simulink model "Predefined_with_GroundTruth_mod1acc"  (R2021b)
settings: Solver=VariableStepAuto  StartTime=0.0  StopTime=inf  RelTol=1e-3
model workspace (MAT data in the model file):
  firstWarning = 1
  originalScenarioChecksum = '114339432DE22364D47BB28FC96DC10C'
undefined symbols (not defined in the file or in its folder): Acceleration, ActorID, AngularVelocity, curvature, curvatureAhd, DefaultGear, DEND_B, DEND_S, DEND_T, direction, driving, gradbp, LF, LR, matlabshared, MAX_BRAKE, MAX_STEER, MAX_TORQUE, MCAR, MIN_BRAKE, MIN_STEER, MIN_TORQUE, NUMD_B, NUMD_S, NUMD_T, Pitch, Position, psi_o, R, Roll, RRdamp, scenario, SceneInfo, sigbuilder_block, STEER_RATIO, stopSign_ID, Tdead, thetaRefs, TL_ID, TrackWidth, Ts, ts, Vdead, Velocity, X_o, xRef2s, Y_o, Yaw, yRef2s
libraries: mpcsigdimcheck_private x10, drivingscenarioandsensors x8, drivingvehiclecontroller x2, slpidlib x2, simulink x2, trackingutilitieslib x2, mpclib x1, simulink_extras x1, drivinglib x1, autolibshared x1, vehdynlibviscommon x1, vehdynlibsteering x1
(part 2 of 3)

== system Predefined_with_GroundTruth_mod1acc/Tracking/Subsystem1 ==
  In2 : Inport
  EgoV : Inport  Port=2
  Camera : drivingscenarioandsensors/Vision Detection Generator  SensorIndex=1  DetectorOutput=Objects only  UpdateInterval=0.1  LaneUpdateInterval=0.1  SensorLocation=[1.9 0]  Height=1.1  Yaw=0  Pitch=1  Roll=0  BusNameSource=Auto  BusName=BusObjectDetections  BusName2Source=Auto  BusName2=BusLaneDetections  MaxNumDetectionsSource=Property  MaxNumDetections=10  MaxNumLanesSource=Property  MaxNumLanes=30  DetectionCoordinates=Ego Cartesian  SimulateUsing=Interpreted execution  MaxRange=150  BoundingBoxAccuracy=5  ProcessNoiseIntensity=5  MaxSpeed=100  MaxAllowedOcclusion=0.5  MinObjectImageSize=[5 5]  DetectionProbability=0.9  FalsePositivesPerImage=0.1  MinLaneImageSize=[20 3]  LaneBoundaryAccuracy=3  HasNoise=on  InitialSeedSource=Repeatable  InitialSeed=0  UsedSeed=0  ActorProfilesSource=From Scenario Reader block  ActorProfilesParameters=driving.internal.ActorProfilesParameters  ActorProfilesExpression=[struct('ActorID',1,'ClassID',1,'Length',4.7,'Width',1.8,'Height',1.4,'OriginOffset',[-1.35 0 0],'MeshVertices',[3.7 0.9 0.857439446366782;3.7 -0.9 0.857439446366782;3.7 -0.9 0.314878892733564;3.7 0.9 0.314878892733564;3.7 0.9 0.857439446366782;2.525 0.9 0.993079584775086;2.525 -0.9 0.993079584775086;3.7 -0.9 0.857439446366782;1.82 0.72 1.4;0.41 0.72 1.4;0.41 -0.72 1.4;1.82 -0.72 1.4;-0.295 0.9 0.993079584775086;-1 0.9 0.857439446366782;-1 -0.9 0.857439446366782;-0.295 -0.9 0.993079584775086;3.7 0.9 0.857439446366782;3.7 0.9 0.314878892733564;2.525 0.9 0.314878892733564;2.525 0.9 0.993079584775086;2.525 0.9 0.993079584775086;2.525 0.9 0.314878892733564;-0.295 0.9 0.314878892733564;-0.295 0.9 0.993079584775086;-0.295 0.9 0.993079584775086;-0.295 0.9 0.314878892733564;-1 0.9 0.355570934256055;-1 0.9 0.857439446366782;2.525 0.9 0.993079584775086;-0.295 0.9 0.993079584775086;0.41 0.72 1.4;1.82 0.72 1.4;3.7 -0.9 0.857439446366782;3.7 -0.9 0.314878892733564;2.525 -0.9 0.314878892733564;2.525 -0.9 0.993079584775086;2.525 -0.9 0.993079584775086;2.525 -0.9 0.314878892733564;-0.295 -0.9 0.314878892733564;-0.295 -0.9 0.993079584775086;-0.295 -0.9 0.993079584775086;-0.295 -0.9 0.314878892733564;-1 -0.9 0.355570934256055;-1 -0.9 0.857439446366782;2.525 -0.9 0.993079584775086;-0.295 -0.9 0.993079584775086;0.41 -0.72 1.4;1.82 -0.72 1.4;-0.295 0.9 0.993079584775086;-0.295 -0.9 0.993079584775086;0.41 -0.72 1.4;0.41 0.72 1.4;2.525 -0.9 0.993079584775086;1.82 -0.72 1.4;1.82 0.72 1.4;2.525 0.9 0.993079584775086;-1 0.9 0.857439446366782;-1 0.9 0.355570934256055;-1 -0.9 0.355570934256055;-1 -0.9 0.857439446366782;3.7 0.9 0.314878892733564;3.7 -0.9 0.314878892733564;-0.295 -0.9 0.314878892733564;-0.295 0.9 0.314878892733564;-0.295 0.9 0.314878892733564;-1 0.9 0.355570934256055;-1 -0.9 0.355570934256055;-0.295 -0.9 0.314878892733564;0 -0.63 0;0 -0.87 0;0.191030206995054 -0.63 0.0601365173421445;0.191030206995054 -0.87 0.0601365173421445;0.309093367795925 -0.63 0.217575963708927;0.309093367795925 -0.87 0.217575963708927;0.309093367795925 -0.63 0.412181821758201;0.309093367795925 -0.87 0.412181821758201;0.191030206995054 -0.63 0.569621268124983;0.191030206995054 -0.87 0.569621268124983;0 -0.63 0.629757785467128;0 -0.87 0.629757785467128;-0.191030206995054 -0.63 0.569621268124983;-0.191030206995054 -0.87 0.569621268124983;-0.309093367795925 -0.63 0.412181821758201;-0.309093367795925 -0.87 0.412181821758201;-0.309093367795925 -0.63 0.217575963708927;-0.309093367795925 -0.87 0.217575963708927;-0.191030206995054 -0.63 0.0601365173421445;-0.191030206995054 -0.87 0.0601365173421445;0 -0.63 0;0 -0.87 0;0 -0.63 0;0.191030206995054 -0.63 0.0601365173421445;0.309093367795925 -0.63 0.217575963708927;0.309093367795925 -0.63 0.412181821758201;0.191030206995054 -0.63 0.569621268124983;0 -0.63 0.629757785467128;-0.191030206995054 -0.63 0.569621268124983;-0.309093367795925 -0.63 0.412181821758201;-0.309093367795925 -0.63 0.217575963708927;-0.191030206995054 -0.63 0.0601365173421445;0 -0.87 0;0.191030206995054 -0.87 0.0601365173421445;0.309093367795925 -0.87 0.217575963708927;0.309093367795925 -0.87 0.412181821758201;0.191030206995054 -0.87 0.569621268124983;0 -0.87 0.629757785467128;-0.191030206995054 -0.87 0.569621268124983;-0.309093367795925 -0.87 0.412181821758201;-0.309093367795925 -0.87 0.217575963708927;-0.191030206995054 -0.87 0.0601365173421445;0 0.87 0;0 0.63 0;0.191030206995054 0.87 0.0601365173421445;0.191030206995054 0.63 0.0601365173421445;0.309093367795925 0.87 0.217575963708927;0.309093367795925 0.63 0.217575963708927;0.309093367795925 0.87 0.412181821758201;0.309093367795925 0.63 0.412181821758201;0.191030206995054 0.87 0.569621268124983;0.191030206995054 0.63 0.569621268124983;0 0.87 0.629757785467128;0 0.63 0.629757785467128;-0.191030206995054 0.87 0.569621268124983;-0.191030206995054 0.63 0.569621268124983;-0.309093367795925 0.87 0.412181821758201;-0.309093367795925 0.63 0.412181821758201;-0.309093367795925 0.87 0.217575963708927;-0.309093367795925 0.63 0.217575963708927;-0.191030206995054 0.87 0.0601365173421445;-0.191030206995054 0.63 0.0601365173421445;0 ...(+3718 chars)],'MeshFaces',[1 2 3;3 4 1;5 6 7;7 8 5;9 10 11;11 12 9;13 14 15;15 16 13;17 18 19;19 20 17;21 22 23;23 24 21;25 26 27;27 28 25;29 30 31;31 32 29;33 34 35;35 36 33;37 38 39;39 40 37;41 42 43;43 44 41;45 46 47;47 48 45;49 50 51;51 52 49;53 54 55;55 56 53;57 58 59;59 60 57;61 62 63;63 64 61;65 66 67;67 68 65;69 71 72;72 70 69;71 73 74;74 72 71;73 75 76;76 74 73;75 77 78;78 76 75;77 79 80;80 78 77;79 81 82;82 80 79;81 83 84;84 82 81;83 85 86;86 84 83;85 87 88;88 86 85;87 89 90;90 88 87;91 92 93;91 93 94;91 94 95;91 95 96;91 96 97;91 97 98;91 98 99;91 99 100;101 102 103;101 103 104;101 104 105;101 105 106;101 106 107;101 107 108;101 108 109;101 109 110;111 113 114;114 112 111;113 115 116;116 114 113;115 117 118;118 116 115;117 119 120;120 118 117;119 121 122;122 120 119;121 123 124;124 122 121;123 125 126;126 124 123;125 127 128;128 126 125;127 129 130;130 128 127;129 131 132;132 130 129;133 134 135;133 135 136;133 136 137;133 137 138;133 138 139;133 139 140;133 140 141;133 141 142;143 144 145;143 145 146;143 146 147;143 147 148;143 148 149;143 149 150;143 150 151;143 151 152;153 155 156;156 154 153;155 157 158;158 156 155;157 159 160;160 158 157;159 161 162;162 160 159;161 163 164;164 162 161;163 165 166;166 164 163;165 167 168;168 166 165;167 169 170;170 168 167;169 171 172;172 170 169;171 173 174;174 172 171;175 176 177;175 177 178;175 178 179;175 179 180;175 180 181;175 181 182;175 182 183;175 183 184;185 186 187;185 187 188;185 188 189;185 189 190;185 190 191;185 191 192;185 192 193;185 193 194;195 197 198;198 196 195;197 199 200;200 198 197;199 201 202;202 200 199;201 203 204;204 202 201;203 205 206;206 204 203;205 207 208;208 206 205;207 209 210;210 208 207;209 211 212;212 210 209;211 213 214;214 212 211;213 215 216;216 214 213;217 218 219;217 219 220;217 220 221;217 221 222;217 222 223;217 223 224;217 224 225;217 225 226;227 228 229;227 229 230;227 230 231;227 231 232;227 232 233;227 233 234;227 234 235;227 235 236],'RCSPattern',[10 10;10 10],'RCSAzimuthAngles',[-180 180],'RCSElevationAngles',[-90 90]); struct('ActorID',2,'ClassID',7,'Length',0.7,'Width',0.2,'Height',0.1,'OriginOffset',[0 0 0],'MeshVertices',[0.35 -0.1 0.1;0.35 0.1 0.1;-0.35 0.1 0.1;-0.35 -0.1 0.1;0.35 -0.1 0;0.35 0.1 0;-0.35 0.1 0;-0.35 -0.1 0],'MeshFaces',[6 2 1;1 5 6;8 4 3;3 7 8;6 7 3;3 2 6;5 1 4;4 8 5;4 1 2;2 3 4;7 6 5;5 8 7],'RCSPattern',[10 10;10 10],'RCSAzimuthAngles',[-180 180],'RCSElevationAngles',[-90 90])]  Intrinsics=driving.internal.cameraIntrinsics('FocalLength',[800 800],'PrincipalPoint',[320 240],'ImageSize',[480 640],'RadialDistortion',[0 0],'TangentialDistortion',[0 0],'Skew',0)
  Detection Concatenation : trackingutilitieslib/Detection Concatenation  NumInputs=3  BusNameSource=Auto  BusName=BusDetectionConcatenation  SimulateUsing=Interpreted execution
      settings: SourceProductBaseCode=AE,DR,TF,RA,UV,VE
  Lidar Point Cloud Generator : drivingscenarioandsensors/Lidar Point Cloud Generator  SensorIndex=2  UpdateInterval=0.1  SensorLocation=[1.5 0]  Height=1.6  Yaw=0  Pitch=0  Roll=0  DetectionCoordinates=Ego Cartesian  HasEgoVehicle=on  EgoVehicleActorID=1  HasRoadsInputPort=on  ActorProfilesSource=From Scenario Reader block  ActorProfilesVariableName=actor_profiles  MaxRange=120  RangeAccuracy=0.002  AzimuthResolution=0.16  ElevationResolution=1.25  AzimuthLimits=[-60 60]  ElevationLimits=[ -20, 20 ]  HasNoise=on
      settings: SourceProductBaseCode=DR
  Lidar Point Cloud Generator1 : drivingscenarioandsensors/Lidar Point Cloud Generator  SensorIndex=3  UpdateInterval=0.1  SensorLocation=[1.5 0]  Height=1.6  Yaw=0  Pitch=0  Roll=0  DetectionCoordinates=Ego Cartesian  HasEgoVehicle=on  EgoVehicleActorID=1  HasRoadsInputPort=on  ActorProfilesSource=From Scenario Reader block  ActorProfilesVariableName=actor_profiles  MaxRange=120  RangeAccuracy=0.002  AzimuthResolution=0.16  ElevationResolution=1.25  AzimuthLimits=[60 180]  ElevationLimits=[ -20, 20 ]  HasNoise=on
      settings: SourceProductBaseCode=DR
  Lidar Point Cloud Generator2 : drivingscenarioandsensors/Lidar Point Cloud Generator  SensorIndex=4  UpdateInterval=0.1  SensorLocation=[1.5 0]  Height=1.6  Yaw=0  Pitch=0  Roll=0  DetectionCoordinates=Ego Cartesian  HasEgoVehicle=on  EgoVehicleActorID=1  HasRoadsInputPort=on  ActorProfilesSource=From Scenario Reader block  ActorProfilesVariableName=actor_profiles  MaxRange=120  RangeAccuracy=0.002  AzimuthResolution=0.16  ElevationResolution=1.25  AzimuthLimits=[-180 -60]  ElevationLimits=[ -20, 20 ]  HasNoise=on
      settings: SourceProductBaseCode=DR
  Camera Detections : Outport
  Radar detections : Outport  Port=2
  wires:
  EgoV/1 -> Lidar Point Cloud Generator1/2, Lidar Point Cloud Generator/2, Lidar Point Cloud Generator2/2
  Lidar Point Cloud Generator1/1 -> Detection Concatenation/2  "Lidar Detections"
  Lidar Point Cloud Generator2/1 -> Detection Concatenation/3  "Lidar Detections"
  Detection Concatenation/1 -> Radar detections/1
  Camera/1 -> Camera Detections/1  "Camera Detections"
  In2/1 -> Camera/1, Lidar Point Cloud Generator/1, Lidar Point Cloud Generator1/1, Lidar Point Cloud Generator2/1
  Lidar Point Cloud Generator/1 -> Detection Concatenation/1  "Lidar Detections"

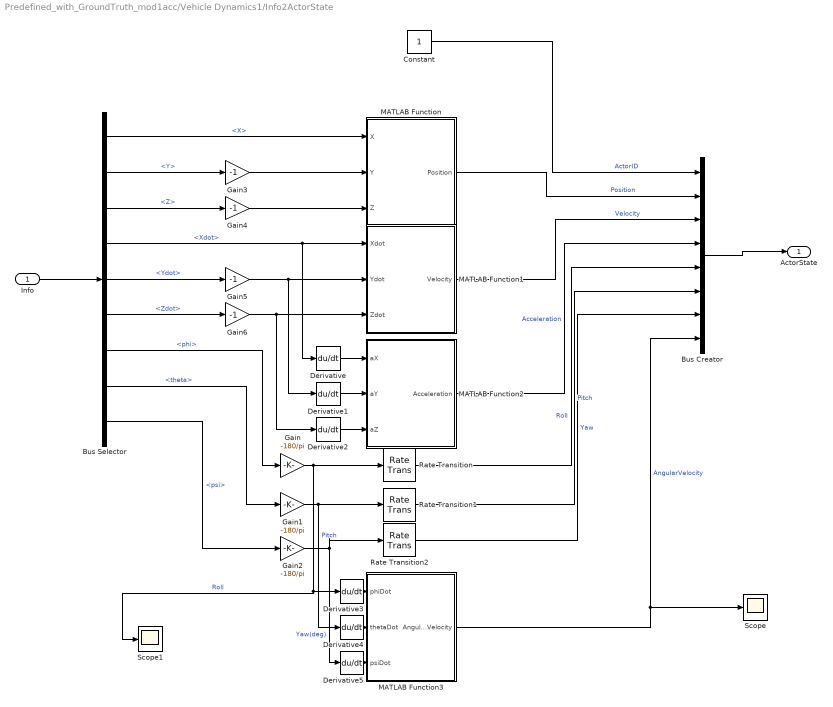
== system Predefined_with_GroundTruth_mod1acc/Vehicle Dynamics1/Info2ActorState ==
  Info : Inport
  Bus Creator : BusCreator  Inputs=ActorID,Position,Velocity,Acceleration,Roll,Pitch,Yaw,AngularVelocity  OutDataTypeStr=Bus: BusActorState  NonVirtualBus=on
  Bus Selector : BusSelector  OutputSignals=InertFrm.Cg.Disp.X,InertFrm.Cg.Disp.Y,InertFrm.Cg.Disp.Z,InertFrm.Cg.Vel.Xdot,InertFrm.Cg.Vel.Ydot,InertFrm.Cg.Vel.Zdot,InertFrm.Cg.Ang.phi,InertFrm.Cg.Ang.theta,InertFrm.Cg.Ang.psi
  Constant : Constant  SampleTime=0.05
  Derivative{,1..5} (6 alike) : Derivative
  Gain : Gain  Gain=-180/pi
  Gain1 : Gain  Gain=-180/pi
  Gain2 : Gain  Gain=-180/pi
  Gain{3..6} (4 alike) : Gain  Gain=-1
  MATLAB Function : MATLAB Function  TreatAsAtomicUnit=on  SystemSampleTime=0.05
  MATLAB Function1 : MATLAB Function  TreatAsAtomicUnit=on  SystemSampleTime=0.05
  MATLAB Function2 : MATLAB Function  TreatAsAtomicUnit=on  SystemSampleTime=0.05
  MATLAB Function3 : MATLAB Function  TreatAsAtomicUnit=on  SystemSampleTime=0.05
  Rate Transition : RateTransition  OutPortSampleTime=0.05
  Rate Transition1 : RateTransition  OutPortSampleTime=0.05
  Rate Transition2 : RateTransition  OutPortSampleTime=0.05
  Scope : Scope
  Scope1 : Scope
  ActorState : Outport
  wires:
  Gain/1 -> Scope1/1, Derivative3/1, Rate Transition/1  "Roll"
  Derivative4/1 -> MATLAB Function3/2(thetaDot)
  Bus Selector/2 -> Gain3/1  "<Y>"
  Bus Selector/4 -> Derivative/1, MATLAB Function1/1(Xdot)  "<Xdot>"
  MATLAB Function1/1(Velocity) -> Bus Creator/3  "Velocity"
  MATLAB Function/1(Position) -> Bus Creator/2  "Position"
  Derivative1/1 -> MATLAB Function2/2(aY)
  Bus Selector/5 -> Gain5/1  "<Ydot>"
  Bus Selector/1 -> MATLAB Function/1(X)  "<X>"
  Bus Selector/9 -> Gain2/1  "<psi>"
  Gain2/1 -> Rate Transition2/1, Derivative5/1  "Yaw(deg)"
  Derivative5/1 -> MATLAB Function3/3(psiDot)
  Bus Selector/7 -> Gain/1  "<phi>"
  MATLAB Function2/1(Acceleration) -> Bus Creator/4  "Acceleration"
  Derivative3/1 -> MATLAB Function3/1(phiDot)
  Gain1/1 -> Derivative4/1, Rate Transition1/1  "Pitch"
  Bus Selector/6 -> Gain6/1  "<Zdot>"
  Bus Selector/8 -> Gain1/1  "<theta>"
  MATLAB Function3/1(AngularVelocity) -> Bus Creator/8, Scope/1  "AngularVelocity"
  Bus Selector/3 -> Gain4/1  "<Z>"
  Derivative2/1 -> MATLAB Function2/3(aZ)
  Derivative/1 -> MATLAB Function2/1(aX)
  Info/1 -> Bus Selector/1
  Constant/1 -> Bus Creator/1  "ActorID"
  Bus Creator/1 -> ActorState/1
  Rate Transition/1 -> Bus Creator/5  "Roll"
  Rate Transition1/1 -> Bus Creator/6  "Pitch"
  Rate Transition2/1 -> Bus Creator/7  "Yaw"
  Gain3/1 -> MATLAB Function/2(Y)
  Gain4/1 -> MATLAB Function/3(Z)
  Gain5/1 -> Derivative1/1, MATLAB Function1/2(Ydot)
  Gain6/1 -> Derivative2/1, MATLAB Function1/3(Zdot)

== system Predefined_with_GroundTruth_mod1acc/Vehicle Dynamics1/Subsystem ==
  Gain : Gain  Gain=MAX_TORQUE*0.1
  Gain1 : Gain  Gain=MIN_BRAKE*0.06
  Gain2 : Gain  Gain=MAX_STEER/4.5
  Signal Builder : Subsystem  Tag=STV Subsys  LoadFcn=sigbuilder_block('load');  StartFcn=sigbuilder_block('start');  StopFcn=sigbuilder_block('stop');  ClipboardFcn=sigbuilder_block('clipboard');  mask(Sigbuilder block){tuvar=[0:10]}
      mask help: Simulink:masks:SigbuilderBlock_MD
      mask init:
      | if ~strcmp(get_param(bdroot(gcbh),'SimulationStatus'),'stopped') tuvar = sigbuilder_block('maskInit'); end
      settings: CopyFcn=sigbuilder_block('copy');  DeleteFcn=sigbuilder_block('delete');  ModelCloseFcn=sigbuilder_block('modelClose');  PreSaveFcn=sigbuilder_block('preSave');  PauseFcn=sigbuilder_block('pause');  ContinueFcn=sigbuilder_block('continue');  NameChangeFcn=sigbuilder_block('namechange');  OpenFcn=sigbuilder_block('open',[0 30 960 455.5 ]);  CloseFcn=sigbuilder_block('close');
      mask Display: plot(0, 0, 100, 100,[2, 2, 32, 32, 2], [68, 8, 8, 68, 68],[32, 2], [38, 38], [32, 19, 2],[53, 60, 44], [32, 17, 17, 2],[16, 16, 31, 31]);txt = getActiveGroup(gcbh);text(2, 100, txt,'verticalAlignment', 'top');
  torque_cmd (Nm) : Outport
  brake_cmd (Nm) : Outport  Port=2
  steer_cmd (deg) : Outport  Port=3
  wires:
  Gain2/1 -> steer_cmd (deg)/1  "steer_cmd (deg)"
  Signal Builder/1(Normalized Torque) -> Gain/1
  Signal Builder/2(Normalized Brake) -> Gain1/1
  Signal Builder/3(Normalized Steer) -> Gain2/1  "steer_cmd (deg)"
  Gain1/1 -> brake_cmd (Nm)/1  "brake_cmd (Nm)"
  Gain/1 -> torque_cmd (Nm)/1  "torque_cmd (Nm)"

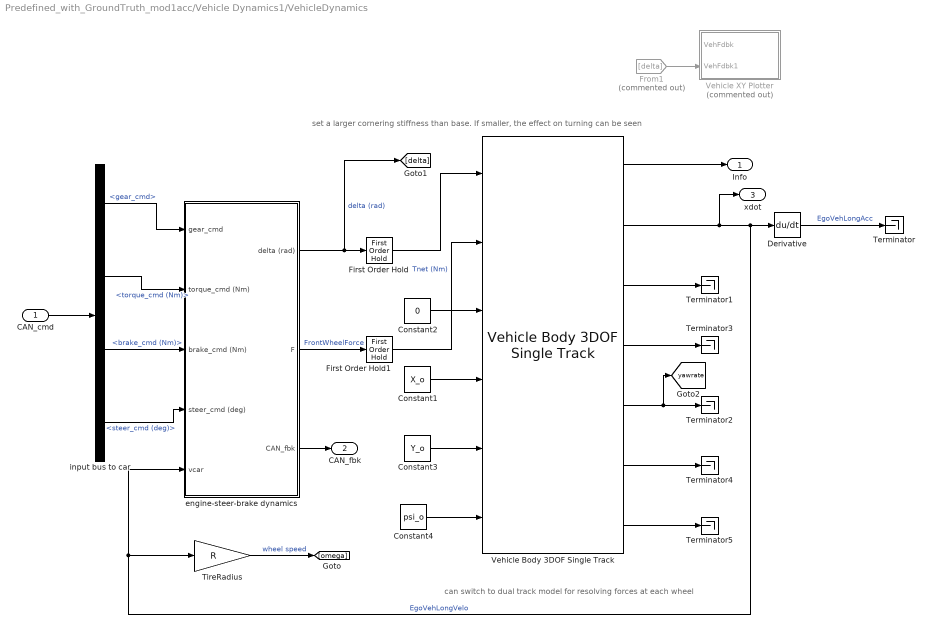
== system Predefined_with_GroundTruth_mod1acc/Vehicle Dynamics1/VehicleDynamics ==
  note: set a larger cornering stiffness than base. If smaller, the effect on turning can be seen
  note: can switch to dual track model for resolving forces at each wheel
  CAN_cmd : Inport
  Constant1 : Constant  Value=X_o
  Constant2 : Constant  Value=0
  Constant3 : Constant  Value=Y_o
  Constant4 : Constant  Value=psi_o
  Derivative : Derivative
  First Order Hold : FirstOrderHold  ErrorTolerance=inf
  First Order Hold1 : FirstOrderHold  ErrorTolerance=inf
  From1 : From  Commented=on  GotoTag=delta
  Terminator{,1..5} (6 alike) : Terminator
  TireRadius : Gain  Gain=R
  Vehicle Body 3DOF Single Track : autolibshared/Vehicle Body 3DOF Single Track  trackMode=Single (bicycle)  inputMode=External longitudinal forces  frontSteerMode=on  rearSteerMode=off  windMode=off  muMode=off  extFMode=off  extMMode=off  htchFMode=off  htchMMode=off  extXo=on  extpsio=on  extxdoto=off  extro=off  extYo=on  extTamb=off  extydoto=off  aMode=2  NF=2  NR=2  m=MCAR  a=LF  b=LR  h=0.35  dh=1  hh=0.2  X_o=InitPosition(1)  xdot_o=InitSpeed  CalphaMode=off  sigmaMode=on  d=0  hl=0  w=[1.4,1.4]  Cy_f=12e3*100  Cy_r=11e3*100  sigma_f=.1  sigma_r=.1  alpha_f_brk=[-.1 .1]  Cy_f_data=[-9e3 9e3]  alpha_r_brk=[-.1 .1]  Cy_r_data=[-9e3 9e3]  Y_o=-InitPosition(2)  ydot_o=0  Izz=2050  psi_o=-InitYaw/180*pi  r_o=0  Af=2  Cd=.3  Cl=.1  Cpm=.1  beta_w=[0:0.01:0.3]  Cs=[0:0.03:0.9]  Cym=[0:0.01:0.3]  Pabs=101325  Tair=273  g=9.81  mu=1  xdot_tol=.01  Fznom=5000  Fxtire_sat=7e4  Fytire_sat=7e4  longOff=0  latOff=0  vertOff=0  wrapAng=off
      settings: SourceProductBaseCode=PW,DR,MT,UV,VE
  Vehicle XY Plotter : Subsystem  Commented=on  mask(Vehicle XY Plotter){a=LF, b=LR, w=TrackWidth, bufferSize=1024, pltDT=.1}
      mask prompts: a "Distance to front axle from CG, a [m]:"; b "Distance to rear axle from CG, b [m]:"; w "Track width, w [m]:"; bufferSize "Path buffer sampe size, bufferSize []:"; pltDT "Plot update rate, pltDT [s]:"
      mask help: This block will display a MATLAB figure which indicates the vehicle path, current position and heading velocity.
      mask TypeOptions a: Vehicle XY Plotter/a
      mask TypeOptions b: Vehicle XY Plotter/b
      mask TypeOptions w: Vehicle XY Plotter/w
      mask TypeOptions bufferSize: Vehicle XY Plotter/bufferSize
  engine-steer-brake dynamics : Subsystem
  input bus to car : BusSelector  OutputSignals=gear_cmd,torque_cmd (Nm),brake_cmd (Nm),steer_cmd (deg)
  Info : Outport
  CAN_fbk : Outport  Port=2  VectorParamsAs1DForOutWhenUnconnected=off
  xdot : Outport  Port=3
  tag scope: yawrate=global
  wires:
  TireRadius/1 -> [omega]  "wheel speed"
  Vehicle Body 3DOF Single Track/1 -> Info/1
  From1/1 -> Vehicle XY Plotter/2(VehFdbk1)
  input bus to car/1 -> engine-steer-brake dynamics/1(gear_cmd)  "<gear_cmd>"
  input bus to car/3 -> engine-steer-brake dynamics/3(brake_cmd (Nm))  "<brake_cmd (Nm)>"
  engine-steer-brake dynamics/1(delta (rad)) -> [delta], First Order Hold/1  "delta (rad)"
  input bus to car/2 -> engine-steer-brake dynamics/2(torque_cmd (Nm))  "<torque_cmd (Nm)>"
  input bus to car/4 -> engine-steer-brake dynamics/4(steer_cmd (deg))  "<steer_cmd (deg)>"
  engine-steer-brake dynamics/3(CAN_fbk) -> CAN_fbk/1
  CAN_cmd/1 -> input bus to car/1
  Constant2/1 -> Vehicle Body 3DOF Single Track/3
  engine-steer-brake dynamics/2(F) -> First Order Hold1/1  "FrontWheelForce"
  First Order Hold/1 -> Vehicle Body 3DOF Single Track/1
  Vehicle Body 3DOF Single Track/2 -> xdot/1, engine-steer-brake dynamics/5(vcar), TireRadius/1, Derivative/1  "EgoVehLongVelo"
  Vehicle Body 3DOF Single Track/3 -> Terminator1/1
  Vehicle Body 3DOF Single Track/4 -> Terminator3/1
  Vehicle Body 3DOF Single Track/5 -> [yawrate], Terminator2/1
  Vehicle Body 3DOF Single Track/6 -> Terminator4/1
  Vehicle Body 3DOF Single Track/7 -> Terminator5/1
  Derivative/1 -> Terminator/1  "EgoVehLongAcc"
  First Order Hold1/1 -> Vehicle Body 3DOF Single Track/2  "Tnet (Nm)"
  Constant1/1 -> Vehicle Body 3DOF Single Track/4
  Constant3/1 -> Vehicle Body 3DOF Single Track/5
  Constant4/1 -> Vehicle Body 3DOF Single Track/6

== system Predefined_with_GroundTruth_mod1acc/Reference Data/Theta/thetaBlocks ==
  note: theta calculated from Simulink blocks
  y : Inport
  x : Inport  Port=2
  dis : Inport  Port=3
  Atan2 : Trigonometry  Operator=atan2  ApproximationMethod=CORDIC
  Difference : simulink/Discrete/Difference  ICPrevInput=0.0  OutMin=[]  OutMax=[]  OutDataType=fixdt(1, 16)  OutScaling=2^-10  DoSatur=off
  Difference1 : simulink/Discrete/Difference  ICPrevInput=0.0  OutMin=[]  OutMax=[]  OutDataType=fixdt(1, 16)  OutScaling=2^-10  DoSatur=off
  IC : InitialCondition  Value=psi_o
  Radians to Degrees : simulink_extras/Transformations/Radians to Degrees
  Terminator : Terminator
  theta : Outport
  wires:
  IC/1 -> Radians to Degrees/1
  Atan2/1 -> IC/1
  dis/1 -> Terminator/1
  x/1 -> Difference1/1
  y/1 -> Difference/1
  Radians to Degrees/1 -> theta/1
  Difference/1 -> Atan2/1
  Difference1/1 -> Atan2/2

== system Predefined_with_GroundTruth_mod1acc/Reference Data/Theta/thetaLt ==
  note: Check out the script "setUpModel" to understand how we have calculated theta
  note: theta based on lookup table
  y : Inport
  x : Inport  Port=2
  dis : Inport  Port=3
  Terminator : Terminator
  Terminator1 : Terminator
  Theta Ref : Lookup_n-D  NumberOfTableDimensions=1  BreakpointsForDimension1=gradbp  Table=thetaRefs  InternalRulePriority=Speed  RndMeth=Simplest  InputSameDT=on
  theta : Outport
  wires:
  Theta Ref/1 -> theta/1
  dis/1 -> Theta Ref/1
  x/1 -> Terminator1/1
  y/1 -> Terminator/1

== system Predefined_with_GroundTruth_mod1acc/Subsystem3/Subsystem1/Subsystem2 ==
  acc_cmd : Inport
  decc_cmd : Inport  Port=2
  Subsystem : Subsystem
  Subsystem1 : Subsystem
  T_eng_cmd : Outport
  brake_cmd : Outport  Port=2
  wires:
  acc_cmd/1 -> Subsystem/1(acc_cmd)
  Subsystem/1(T_eng_cmd) -> T_eng_cmd/1
  decc_cmd/1 -> Subsystem1/1(decc_cmd)
  Subsystem1/1(T_brake_cmd) -> brake_cmd/1

== system Predefined_with_GroundTruth_mod1acc/Subsystem3/Subsystem2/Subsystem2 ==
  acc_cmd : Inport
  decc_cmd : Inport  Port=2
  Subsystem : Subsystem
  Subsystem1 : Subsystem
  T_eng_cmd : Outport
  brake_cmd : Outport  Port=2
  wires:
  acc_cmd/1 -> Subsystem/1(acc_cmd)
  Subsystem/1(T_eng_cmd) -> T_eng_cmd/1
  decc_cmd/1 -> Subsystem1/1(decc_cmd)
  Subsystem1/1(T_brake_cmd) -> brake_cmd/1

== system Predefined_with_GroundTruth_mod1acc/Vehicle Dynamics1/Subsystem/Signal Builder ==
  Demux : Demux  Tag=STV Demux  Outputs=3
      settings: DisplayOption=none
  FromWs : FromWorkspace  Tag=STV FromWs  VariableName=tuvar
      SigBuilderData=|
      | common.afterFinalStr = 'Extrapolate'
      | common.sampleTime = 0
      | dataSet.timeRange = [0 3.5]
      | dataSet.name = 'DriveAndTurn'
      | sbobj.Groups.Name = 'DriveAndTurn'
      | sbobj.Groups.Signals(1).Name = 'Normalized Torque'
      | sbobj.Groups.Signals(1).XData = [0 1 1 2 2 3.5]
      | sbobj.Groups.Signals(1).YData = [1 1 0 0 1 1]
      | sbobj.Groups.Signals(2).Name = 'Normalized Brake'
      | sbobj.Groups.Signals(2).XData = [0 1 1 2 2 3.5]
      | sbobj.Groups.Signals(2).YData = [0 0 1 1 0 0]
      | sbobj.Groups.Signals(3).Name = 'Normalized Steer'
      | sbobj.Groups.Signals(3).XData = [0 0.5 0.6 1.02 1.02 2 2.5 3 3.5]
      | sbobj.Groups.Signals(3).YData = [-0.02 -0.02 -0.02 -0.3 -1.02 -0.92 -0.34 0.14 0.22]
      | sbobj.Groups.TimeRange = [0 3.5]
  Normalized Torque : Outport  Tag=STV Outport
  Normalized Brake : Outport  Tag=STV Outport  Port=2
  Normalized Steer : Outport  Tag=STV Outport  Port=3
  wires:
  FromWs/1 -> Demux/1
  Demux/1 -> Normalized Torque/1
  Demux/2 -> Normalized Brake/1
  Demux/3 -> Normalized Steer/1

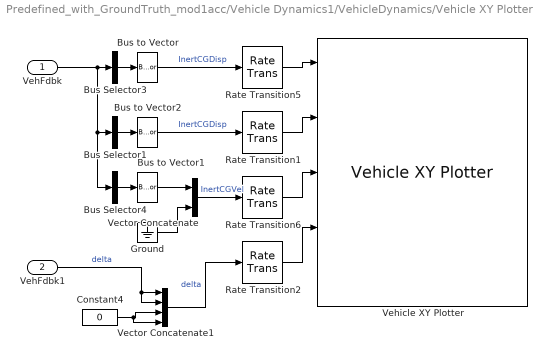
== system Predefined_with_GroundTruth_mod1acc/Vehicle Dynamics1/VehicleDynamics/Vehicle XY Plotter ==
  VehFdbk : Inport
  VehFdbk1 : Inport  Port=2
  Bus Selector1 : BusSelector  OutputSignals=InertFrm.Cg.Ang.phi,InertFrm.Cg.Ang.theta,InertFrm.Cg.Ang.psi  OutputAsBus=on
  Bus Selector3 : BusSelector  OutputSignals=InertFrm.Geom.Disp.X,InertFrm.Geom.Disp.Y,InertFrm.Geom.Disp.Z  OutputAsBus=on
  Bus Selector4 : BusSelector  OutputSignals=InertFrm.Cg.Vel.Xdot,InertFrm.Cg.Vel.Ydot  OutputAsBus=on
  Bus to Vector : BusToVector
  Bus to Vector1 : BusToVector
  Bus to Vector2 : BusToVector
  Constant4 : Constant  Value=0
  Ground : Ground
  Rate Transition{1..2,5..6} (4 alike) : RateTransition  OutPortSampleTime=pltDT
  Vector Concatenate : Concatenate
  Vector Concatenate1 : Concatenate  NumInputs=4
  Vehicle XY Plotter : vehdynlibviscommon/Vehicle XY Plotter  w=w  a=a  b=b  figBorder=2000  bufferSize=bufferSize  extStats=off  extTireF=off
      settings: SourceProductName=The database C:\Users\jrodgers\AppData\Roaming\MathWorks\MATLAB\R2018b\slblocks_master.db is locked, or a table in the database is locked. (database is locked)
  wires:
  Bus to Vector2/1 -> Rate Transition1/1  "InertCGDisp"
  Rate Transition5/1 -> Vehicle XY Plotter/1
  Bus Selector4/1 -> Bus to Vector1/1
  Rate Transition1/1 -> Vehicle XY Plotter/2
  Rate Transition6/1 -> Vehicle XY Plotter/3
  Vector Concatenate/1 -> Rate Transition6/1  "InertCGVel"
  Bus Selector1/1 -> Bus to Vector2/1
  Bus to Vector/1 -> Rate Transition5/1  "InertCGDisp"
  Bus Selector3/1 -> Bus to Vector/1
  Bus to Vector1/1 -> Vector Concatenate/1
  Ground/1 -> Vector Concatenate/2
  VehFdbk/1 -> Bus Selector1/1, Bus Selector4/1, Bus Selector3/1
  Rate Transition2/1 -> Vehicle XY Plotter/4
  Constant4/1 -> Vector Concatenate1/4, Vector Concatenate1/3
  VehFdbk1/1 -> Vector Concatenate1/2, Vector Concatenate1/1  "delta"
  Vector Concatenate1/1 -> Rate Transition2/1  "delta"

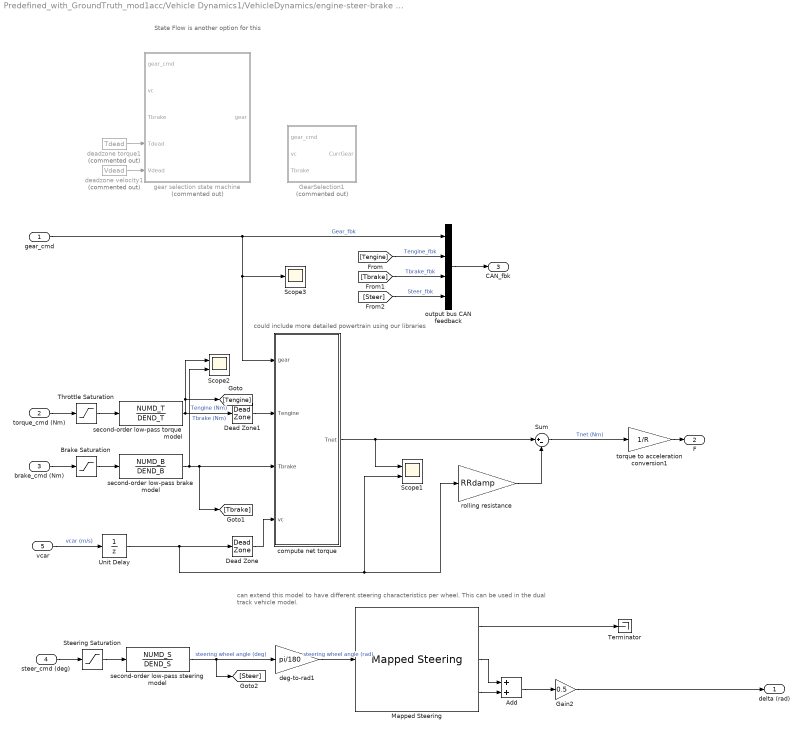
== system Predefined_with_GroundTruth_mod1acc/Vehicle Dynamics1/VehicleDynamics/engine-steer-brake dynamics ==
  note: State Flow is another option for this
  note: could include more detailed powertrain using our libraries
  note: can extend this model to have different steering characteristics per wheel. This can be used in the dual track vehicle model.
  gear_cmd : Inport
  torque_cmd (Nm) : Inport  Port=2
  brake_cmd (Nm) : Inport  Port=3
  steer_cmd (deg) : Inport  Port=4
  vcar : Inport  Port=5
  Add : Sum
  Brake Saturation : Saturate  UpperLimit=MAX_BRAKE  LowerLimit=MIN_BRAKE
  Dead Zone : DeadZone  LowerValue=-Vdead  UpperValue=Vdead  SaturateOnIntegerOverflow=on
  Dead Zone1 : DeadZone  LowerValue=-Tdead  UpperValue=Tdead  SaturateOnIntegerOverflow=on
  Gain2 : Gain  Gain=0.5
  GearSelection1 : Stateflow chart  Commented=on  TreatAsAtomicUnit=on  SystemSampleTime=ts
      settings: PortSchema="{\"entries\":[{\"content\":{\"sides\":[{\"content\":{\"connectorIds\":[\"In3\",\"In2\",\"In1\"]},\"type\":\"ConnectorPlacement.EquallySpacedRectSide\",\"uuid\":\"465e5722-891f-481b-b3b6-2b8339e8e743\"},{\"content\":{\"connectorIds\":[\"Out1\"],\"side\":\"RIGHT\"},\"type\":\"ConnectorPlacement.EquallySpacedRectSide\",\"uuid\":\"28ef13cd-41d9-4e2e-8cd9-9157abf573a9\"},{\"content\":{\"connectorIds\":[],\"side\":\"TOP\"},\"type\":\"ConnectorPlacement.EquallySpacedRectSide\",\"uuid\":\"44f19923-60ae-466f-ad2a-756f1033b52e\"},{\"content\":{\"connectorIds\":[],\"side\":\"HIDDEN\"},\"type\":\"ConnectorPlacement.EquallySpacedRectSide\",\"uuid\":\"d5a146f0-4328-42be-94e3-09f51634e7da\"}]},\"type\":\"ConnectorPlacement.EquallySpacedConnector\",\"uuid\":\"14e271af-3da2-4f7d-9688-fcc3c9792006\"}],\"packageUris\":[\"http://schema.mathworks.com/mf0/Connector/R2020b\"],\"version\":\"1.0\"}"
  Mapped Steering : vehdynlibsteering/Mapped Steering  SpdDpd=off  StrgAngBpts=[-1.5*pi 1.5*pi]  WhlLftTbl=[-1.5*pi 1.5*pi]*STEER_RATIO  WhlRghtTbl=[-1.5*pi 1.5*pi]*STEER_RATIO  VehSpdBpts=[-1 1]  SpdFctTbl=[1 1]  aMode=2
      settings: SourceProductBaseCode=VE
  Scope1 : Scope  NumInputPorts=2
  Scope2 : Scope  NumInputPorts=2
  Scope3 : Scope
  Steering Saturation : Saturate  UpperLimit=MAX_STEER  LowerLimit=MIN_STEER
  Sum : Sum  Inputs=|+-
  Terminator : Terminator
  Throttle Saturation : Saturate  UpperLimit=MAX_TORQUE  LowerLimit=MIN_TORQUE
  Unit Delay : UnitDelay  SampleTime=-1  HasFrameUpgradeWarning=on
  compute net torque : MATLAB Function  TreatAsAtomicUnit=on  SystemSampleTime=ts
  deadzone torque1 : Constant  Commented=on  Value=Tdead  SampleTime=ts
  deadzone velocity1 : Constant  Commented=on  Value=Vdead  SampleTime=ts
  deg-to-rad1 : Gain  Gain=pi/180
  gear selection state machine : MATLAB Function  Commented=on  TreatAsAtomicUnit=on  SystemSampleTime=ts
  output bus CAN feedback : BusCreator  Inputs=4
  rolling resistance : Gain  Gain=RRdamp
  second-order low-pass brake model : DiscreteTransferFcn  Numerator=NUMD_B  Denominator=DEND_B  SampleTime=ts
  second-order low-pass steering model : DiscreteTransferFcn  Numerator=NUMD_S  Denominator=DEND_S  SampleTime=ts
  second-order low-pass torque model : DiscreteTransferFcn  Numerator=NUMD_T  Denominator=DEND_T  SampleTime=ts
  torque to acceleration conversion1 : Gain  Gain=1/R
  delta (rad) : Outport  VectorParamsAs1DForOutWhenUnconnected=off
  F : Outport  Port=2  VectorParamsAs1DForOutWhenUnconnected=off
  CAN_fbk : Outport  Port=3  VectorParamsAs1DForOutWhenUnconnected=off
  wires:
  steer_cmd (deg)/1 -> Steering Saturation/1
  torque_cmd (Nm)/1 -> Throttle Saturation/1
  brake_cmd (Nm)/1 -> Brake Saturation/1
  second-order low-pass steering model/1 -> deg-to-rad1/1, [Steer]  "steering wheel angle (deg)"
  Throttle Saturation/1 -> second-order low-pass torque model/1
  Brake Saturation/1 -> second-order low-pass brake model/1
  Steering Saturation/1 -> second-order low-pass steering model/1
  vcar/1 -> Unit Delay/1  "vcar (m/s)"
  second-order low-pass brake model/1 -> [Tbrake], compute net torque/3(Tbrake), Scope2/2  "Tbrake (Nm)"
  second-order low-pass torque model/1 -> Dead Zone1/1, [Tengine], Scope2/1  "Tengine (Nm)"
  compute net torque/1(Tnet) -> Scope1/1, Sum/1
  rolling resistance/1 -> Sum/2
  deadzone velocity1/1 -> gear selection state machine/5(Vdead)
  deadzone torque1/1 -> gear selection state machine/4(Tdead)
  gear_cmd/1 -> output bus CAN feedback/1, Scope3/1, compute net torque/1(gear)  "Gear_fbk"
  output bus CAN feedback/1 -> CAN_fbk/1
  [Tengine] -> output bus CAN feedback/2  "Tengine_fbk"
  [Tbrake] -> output bus CAN feedback/3  "Tbrake_fbk"
  [Steer] -> output bus CAN feedback/4  "Steer_fbk"
  Mapped Steering/2 -> Add/1
  Mapped Steering/3 -> Add/2
  Add/1 -> Gain2/1
  torque to acceleration conversion1/1 -> F/1
  Mapped Steering/1 -> Terminator/1
  deg-to-rad1/1 -> Mapped Steering/1  "steering wheel angle (rad)"
  Sum/1 -> torque to acceleration conversion1/1  "Tnet (Nm)"
  Dead Zone/1 -> compute net torque/4(vc)
  Dead Zone1/1 -> compute net torque/2(Tengine)
  Unit Delay/1 -> Scope1/2, rolling resistance/1, Dead Zone/1
  Gain2/1 -> delta (rad)/1

== system Predefined_with_GroundTruth_mod1acc/Subsystem3/Subsystem1/Subsystem2/Subsystem ==
  acc_cmd : Inport
  Constant1 : Constant  Value=MCAR
  Gain : Gain  Gain=1.1*MCAR
  Gain1 : Gain  Gain=1.2*0.3*2/2
  Gain2 : Gain  Gain=0.7*9.81
  Gain4 : Gain  Gain=R/(7.05*0.8)
  Integrator : Integrator  ExternalReset=falling
  Square : Math  Operator=square  SaturateOnIntegerOverflow=on
  Sum : Sum  Inputs=+++
  T_eng_cmd : Outport
  wires:
  Constant1/1 -> Gain2/1
  Gain/1 -> Sum/3
  Sum/1 -> Gain4/1
  acc_cmd/1 -> Gain/1, Integrator/2, Integrator/1
  Gain2/1 -> Sum/2
  Gain1/1 -> Sum/1  "F_aero"
  Gain4/1 -> T_eng_cmd/1  "T_eng"
  Integrator/1 -> Square/1  "v"
  Square/1 -> Gain1/1

== system Predefined_with_GroundTruth_mod1acc/Subsystem3/Subsystem1/Subsystem2/Subsystem1 ==
  decc_cmd : Inport
  Constant1 : Constant  Value=MCAR
  Gain : Gain  Gain=1.1*MCAR
  Gain1 : Gain  Gain=1.2*0.3*2/2
  Gain2 : Gain  Gain=0.7*9.81
  Gain4 : Gain  Gain=-R/(7.05*0.8)
  Integrator : Integrator  ExternalReset=falling
  Square : Math  Operator=square  SaturateOnIntegerOverflow=on
  Sum : Sum  Inputs=+++
  T_brake_cmd : Outport
  wires:
  Square/1 -> Gain1/1
  Integrator/1 -> Square/1  "v"
  Gain4/1 -> T_brake_cmd/1  "T_eng"
  Gain1/1 -> Sum/1  "F_aero"
  Gain2/1 -> Sum/2
  decc_cmd/1 -> Integrator/2, Integrator/1, Gain/1
  Sum/1 -> Gain4/1
  Gain/1 -> Sum/3
  Constant1/1 -> Gain2/1

== system Predefined_with_GroundTruth_mod1acc/Subsystem3/Subsystem2/Subsystem2/Subsystem ==
  acc_cmd : Inport
  Constant1 : Constant  Value=MCAR
  Gain : Gain  Gain=1.1*MCAR
  Gain1 : Gain  Gain=1.2*0.3*2/2
  Gain2 : Gain  Gain=0.7*9.81
  Gain4 : Gain  Gain=R/(7.05*0.8)
  Integrator : Integrator  ExternalReset=falling
  Square : Math  Operator=square  SaturateOnIntegerOverflow=on
  Sum : Sum  Inputs=+++
  T_eng_cmd : Outport
  wires:
  Constant1/1 -> Gain2/1
  Gain/1 -> Sum/3
  Sum/1 -> Gain4/1
  acc_cmd/1 -> Gain/1, Integrator/2, Integrator/1
  Gain2/1 -> Sum/2
  Gain1/1 -> Sum/1  "F_aero"
  Gain4/1 -> T_eng_cmd/1  "T_eng"
  Integrator/1 -> Square/1  "v"
  Square/1 -> Gain1/1

== system Predefined_with_GroundTruth_mod1acc/Subsystem3/Subsystem2/Subsystem2/Subsystem1 ==
  decc_cmd : Inport
  Constant1 : Constant  Value=MCAR
  Gain : Gain  Gain=1.1*MCAR
  Gain1 : Gain  Gain=1.2*0.3*2/2
  Gain2 : Gain  Gain=0.7*9.81
  Gain4 : Gain  Gain=-R/(7.05*0.8)
  Integrator : Integrator  ExternalReset=falling
  Square : Math  Operator=square  SaturateOnIntegerOverflow=on
  Sum : Sum  Inputs=+++
  T_brake_cmd : Outport
  wires:
  Square/1 -> Gain1/1
  Integrator/1 -> Square/1  "v"
  Gain4/1 -> T_brake_cmd/1  "T_eng"
  Gain1/1 -> Sum/1  "F_aero"
  Gain2/1 -> Sum/2
  decc_cmd/1 -> Integrator/2, Integrator/1, Gain/1
  Sum/1 -> Gain4/1
  Gain/1 -> Sum/3
  Constant1/1 -> Gain2/1

== matlab function Predefined_with_GroundTruth_mod1acc/Positions and States /MATLAB Function2 ==
  data: Actors input; ss_poses output; ss_State input

function ss_poses = findssposes(Actors, ss_State)

n=length(ss_State);
ss_poses=zeros(n,4);
indices=zeros(n,1);
ID=zeros(length(Actors),1);

for i=1:length(Actors)
 ID(i)=Actors(i).ActorID;
end

indices=find(ismember(ID,ss_State));
if(~isempty(indices))
    
    for i=1:n
        ss_poses(i,:)=([Actors(indices(i)).Position(:)',ss_State(i)]);
    end
end

ss_poses(ss_poses==0)=NaN;






% ss1_poses=zeros(1,4);
% ss2_poses=zeros(1,4);
% for i=1:length(Actors)
%     ID=Actors(i).ActorID;
%     
%     if(ID==ss1_State(1))
%         ss1_poses=[Actors(i).Position(:)',ss1_State(1)];
%     elseif ID== (ss1_State(2))
%         ss2_poses=[Actors(i).Position(:)',ss1_State(2)];
%     
%     end
%   
% end
% ss1_poses(ss1_poses==0)=NaN;   
% ss2_poses(ss2_poses==0)=NaN;

== matlab function Predefined_with_GroundTruth_mod1acc/Positions and States /MATLAB Function1 ==
  data: Actors input; TL_poses output; TL_State input

function TL_poses = findTLposes(Actors, TL_State)
n=length(TL_State);
TL_poses=zeros(n/2,5);
indices=zeros(n/2,1);
ID=zeros(length(Actors),1);

for i=1:length(Actors)
 ID(i)=Actors(i).ActorID;
end

indices=find(ismember(ID,TL_State(n/2+1:end)));
if (~isempty(indices))

    for i=1:n/2
        TL_poses(i,:)=([Actors(indices(i)).Position(:)',TL_State(i),ID(indices(i))]);

    end
end
TL_poses(TL_poses==0)=NaN;

== stateflow chart Predefined_with_GroundTruth_mod1acc/Positions and States /Traffic Light Sensor/Traffic Light Switching Logic ==
  state STEADYRED
    entry:
    trafficLight(:)= Red; TL_ID=TL_id;
  state STEADYGREEN
    entry:
    trafficLight(:)= Green; TL_ID=TL_id;
  state START
    entry:
    trafficLight=TL_id;
    trafficLight(:)= Black;TL_ID=TL_id;
  state TRAFFICLIGHT_ODDYELLOW_EVENRED
    entry:
    trafficLight(1:2:end)=Yellow;TL_ID(1:2:end)=TL_id(1:2:end);
    trafficLight(2:2:end) = Red;TL_ID(2:2:end)=TL_id(2:2:end);
  state TRAFFICLIGHT_ODDGREEN_EVENRED
    entry:
    trafficLight(1:2:end)=Green;TL_ID(1:2:end)=TL_id(1:2:end);
    trafficLight(2:2:end) = Red;TL_ID(2:2:end)=TL_id(2:2:end);
  state TRAFFICLIGHT_ODDRED_EVENYELLOW
    entry:
    trafficLight(1:2:end)=Red;TL_ID(1:2:end)=TL_id(1:2:end);
    trafficLight(2:2:end) = Yellow;TL_ID(2:2:end)=TL_id(2:2:end);
  state TRAFFICLIGHT_ODDRED_EVENGREEN
    entry:
    trafficLight(1:2:end)=Red;TL_ID(1:2:end)=TL_id(1:2:end);
    trafficLight(2:2:end) = Green;TL_ID(2:2:end)=TL_id(2:2:end);
  (default) -> START
  START -> STEADYGREEN [order 3] : [LightConfig==1]
  START -> STEADYRED [order 1] : [LightConfig==2]
  START -> TRAFFICLIGHT_ODDGREEN_EVENRED [order 2] : [LightConfig ==3]
  TRAFFICLIGHT_ODDGREEN_EVENRED -> TRAFFICLIGHT_ODDYELLOW_EVENRED : after(4,sec)
  TRAFFICLIGHT_ODDYELLOW_EVENRED -> TRAFFICLIGHT_ODDRED_EVENGREEN : after(1,sec)
  TRAFFICLIGHT_ODDRED_EVENYELLOW -> TRAFFICLIGHT_ODDGREEN_EVENRED : after(1,sec)
  TRAFFICLIGHT_ODDRED_EVENGREEN -> TRAFFICLIGHT_ODDRED_EVENYELLOW : after(4,sec)
  data: Green constant double =3; Red constant double =1; Yellow constant double =2; LightConfig input; TL_id input; Black constant double =0; TL_ID output; trafficLight output

== matlab function Predefined_with_GroundTruth_mod1acc/MATLAB Function ==
  data: D2S input; Tracking input; ObjectID output; TracksNum output; ObjRelVel output; ObjectDist output; ObjAhead output
function [ObjectID,TracksNum,ObjRelVel,ObjectDist,ObjAhead]= SFDetections(D2S, Tracking)
ObjectID = zeros(20,1);
TrackPos = zeros(3,20);
TrackVel = zeros(3,20);
ObjectDist = 100; % zeros(20,1);
ObjRelVel = 10;
ObjAhead = 0;
TracksNum = Tracking.NumTracks;

for t = 1:TracksNum
    ObjectID(t) = Tracking.Tracks(t).ObjectClassID;
    TrackPos(:,t) = Tracking.Tracks(t).State(1:2:5);
    TrackVel(:,t) = Tracking.Tracks(t).State(2:2:6);

    if abs(TrackPos(2,t)) < 1 && abs(TrackPos(1,t)) < D2S
        ObjAhead = 1;
        ObjectDist = min(ObjectDist,TrackPos(1,t));
        if TrackPos(1,t) <= ObjectDist
            ObjRelVel = TrackVel(1,t);
        end
    end
    
end

== matlab function Predefined_with_GroundTruth_mod1acc/Vehicle Dynamics1/Info2ActorState/MATLAB Function ==
  data: X input; Position output; Y input; Z input
function Position = fcn(X, Y, Z)

Position = [X Y, Z];

== stateflow chart Predefined_with_GroundTruth_mod1acc/Routing ==
  settings: updateMethod=DISCRETE  sampleTime=Ts
  state InitialRoute
    en:
    NewRoute = 0;
  state Rerouting
    en:
    NewRoute = 1;
  (default) -> InitialRoute
  InitialRoute -> Rerouting : [ReRoute == 1]
  Rerouting -> InitialRoute : [ReRoute == 0]
  data: ReRoute input; NewRoute output

== matlab function Predefined_with_GroundTruth_mod1acc/MATLAB Function1 ==
  data: EVpos input; yaw input; Scene output; SceneInfo input; SDir output; SDist input; D2S output; angl output
function [Scene,SDir,D2S,angl] = ScenarioFinder(EVpos,yaw, SceneInfo, SDist)

    % dist = zeros(1,length(SceneLocations));
    for j = 1:length(SceneInfo(:,1))
        distXY = SceneInfo(j,1:2) - EVpos(1:2);
        D2S = norm(distXY);
        
        if (D2S <= SDist)
            Scene = SceneInfo(j,3);
            angl = atan2d(distXY(2),distXY(1));
            angl = angl - yaw;
%             rot = [cosd(angl) -sind(angl);sind(angl) cosd(angl)];
%             distXY = rot*distXY';
%             angl = atan2d(distXY(2),distXY(1));
            
            if angl < 0
                angl = angl + 360;
            end

            if (angl > 315) || (angl <= 45) 
                SDir = "N";
            elseif (angl > 225) && (angl <= 315)
                SDir = "E";
            elseif (angl > 135) && (angl <= 225)
                SDir = "S";
                D2S = 1000;
                angl = 1000;
                Scene = 0;
            elseif (angl > 45) && (angl <= 135)
                SDir = "W";
            else
                SDir = "Error";
            end
            break
        else
            Scene = 0;
            SDir = " ";
            angl = 1000;
            D2S = 1000;
        end

    end

== stateflow chart Predefined_with_GroundTruth_mod1acc/Emergency Stop ==
  settings: updateMethod=DISCRETE  sampleTime=Ts
  state EmergencyCheck
    en:
    EStop = 0;
  state Pullover
    en:
    EStop=1;
  state Stop
    en:
    EStop=2;
  Pullover -> EmergencyCheck : [TechFailure == 0]
  (default) -> EmergencyCheck
  EmergencyCheck -> Pullover [order 1] : [TechFailure == 1]
  EmergencyCheck -> Stop [order 2] : [D2O<=1]
  Stop -> EmergencyCheck : [D2O > 2]
  data: D2O input; TechFailure input; EStop output

== stateflow chart Predefined_with_GroundTruth_mod1acc/Collision Avoidance ==
  settings: sampleTime=ts
  state Start
    en:
    Stuck = 0;
    ACC = 0;
    LaneChangeCmd = 0;
    %VelCmd = CurrentVelCmd;
  state Follow
    en:
    ACC = 1;
  state LaneChange
    en:
    LaneChangeCmd = 1;
  LaneChange -> Start : [LaneChanged == 1]
  (default) -> Start
  Follow -> LaneChange [order 2] : [LaneAvailable == 1 && Stuck == 1]
  Start -> Follow : [ObjAhead == 1]
  Follow -> Start [order 3] : [ObjAhead == 0]
  Follow -> Follow [order 1] : [(EgoSpeed <= MinSpeed) && after(WaitTime,sec)]{Stuck = 1;}
  data: Stuck local; ACC output; WaitTime input; ObjAhead input; MinSpeed input; LaneAvailable input; EgoSpeed input; LaneChanged input; LaneChangeCmd output

== matlab function Predefined_with_GroundTruth_mod1acc/Subsystem3/Subsystem2/MATLAB Function ==
  data: u input; accel output; decel output
function [accel, decel] = fcn(u)
if(u>0)
    accel=u; decel=0;
elseif(u<0)
    accel=0; decel=-u;
else
    accel=0;decel=0;
end

== matlab function Predefined_with_GroundTruth_mod1acc/MATLAB Function2 ==
  data: v input; RefVelCmd output; curvature input
function RefVelCmd = fcn(v,curvature)

    if abs(curvature) >= 0 && abs(curvature) <= 1e-2
        RefVelCmd = v;
    else
        r = 1/abs(curvature);
        RefVelCmd = min(v,sqrt(9.81*r*.7));
    end

== matlab function Predefined_with_GroundTruth_mod1acc/Vehicle Dynamics1/Info2ActorState/MATLAB Function1 ==
  data: Xdot input; Velocity output; Ydot input; Zdot input
function Velocity = fcn(Xdot, Ydot, Zdot)

Velocity = [Xdot Ydot, Zdot];

== matlab function Predefined_with_GroundTruth_mod1acc/Vehicle Dynamics1/Info2ActorState/MATLAB Function2 ==
  data: aX input; Acceleration output; aY input; aZ input
function Acceleration = fcn(aX, aY, aZ)

Acceleration = [aX aY, aZ];

== matlab function Predefined_with_GroundTruth_mod1acc/Vehicle Dynamics1/Info2ActorState/MATLAB Function3 ==
  data: phiDot input; AngularVelocity output; thetaDot input; psiDot input
function AngularVelocity = fcn(phiDot, thetaDot, psiDot)

AngularVelocity = [phiDot thetaDot, psiDot];

== stateflow chart Predefined_with_GroundTruth_mod1acc/Vehicle Dynamics1/VehicleDynamics/engine-steer-brake dynamics/GearSelection1 ==
  state Park
    CurrGear = 0;
  state Reverse
    CurrGear = -1;
  state drive
    CurrGear = 1;
  (default) -> (junction 12)
  (junction 12) -> Reverse [order 3] : [DefaultGear == -1]
  (junction 12) -> drive [order 2] : [DefaultGear == 1]
  (junction 12) -> Park [order 1] : [DefaultGear == 0]
  (junction 12) -> Park [order 4] : %fallback to park
  drive -> Park [order 2] : [gear_cmd == 0 && allowShift(vc,Tbrake)]
  Park -> Reverse [order 2] : [gear_cmd == -1 && allowShift(vc,Tbrake)]
  Park -> drive [order 1] : [gear_cmd == 1 && allowShift(vc,Tbrake)]
  Reverse -> Park [order 2] : [gear_cmd == 0 && allowShift(vc,Tbrake)]
  drive -> Reverse [order 1] : [gear_cmd == -1 && allowShift(vc,Tbrake)]
  Reverse -> drive [order 1] : [gear_cmd == 1 && allowShift(vc,Tbrake)]
  data: Tdead parameter; Vdead parameter; vel function_input; brakeT function_input; allow function_output; CurrGear output; Tbrake input; vc input; gear_cmd input; DefaultGear parameter
  function allow = allowShift(vel, brakeT):
    | function allow = allowShift(vel, brakeT)
    | allow = (abs(vel) <= Vdead) && (abs(brakeT)>Tdead);
    | end

== matlab function Predefined_with_GroundTruth_mod1acc/Vehicle Dynamics1/VehicleDynamics/engine-steer-brake dynamics/compute net torque ==
  data: gear input; Tnet output; Tengine input; Tbrake input; vc input
function Tnet  = net_torque(gear,Tengine,Tbrake,vc)

%  --set engine torque based on current gear selection

if (gear == 0)
    %  --vehicle is in PARK, so force engine torque to zero
    Tengine = 0;
end

Tnet = Tengine + Tbrake*tanh(5*vc);

end

== matlab function Predefined_with_GroundTruth_mod1acc/Vehicle Dynamics1/VehicleDynamics/engine-steer-brake dynamics/gear selection state machine ==
  data: gear output; gear_cmd input; vc input; Tbrake input; Tdead input; Vdead input
function gear = gear_change_FSM(gear_cmd,vc,Tbrake,Tdead,Vdead)

persistent GEAR

%  The vehicle gear can take on one of the following enumerated values:
%  -1 = REVERSE
%   0 = PARK
%   1 = DRIVE

%  --initialize the local persistent variables

if isempty(GEAR)
    %  --default gear at startup is PARK
    %  Note:  Change this to 1 if you want car to initialize in DRIVE
    GEAR = 0;
end


%  --evaluate the gear change finite state machine

switch GEAR
    case 0  % vehicle is in PARK
        if (gear_cmd == 1)
            %  --check to see if we can shift to DRIVE
            if ((abs(vc) <= Vdead) && (abs(Tbrake) > Tdead))
                %  --shift to DRIVE
                GEAR = 1;
            end
            
        elseif (gear_cmd == 2)
            %  --check to see if we can shift to REVERSE
            if ((abs(vc) <= Vdead) && (abs(Tbrake) > Tdead))
                %  --shift to REVERSE
                GEAR = 2;
            end
        end
        
    case 1  % vehicle is in DRIVE
        if (gear_cmd == 0)
            %  --check to see if we can shift to PARK
            if ((abs(vc) <= Vdead) && (abs(Tbrake) > Tdead))
                %  --shift to PARK
                GEAR = 0;
            end
            
        elseif (gear_cmd == 2)
            %  --check to see if we can shift to REVERSE
            if ((abs(vc) <= Vdead) && (abs(Tbrake) > Tdead))
                %  --shift to REVERSE
                GEAR = 2;
            end
        end
        
    case -1  % vehicle is in REVERSE
        if (gear_cmd == 0)
            %  --check to see if we can shift to PARK
            if ((abs(vc) <= Vdead) && (abs(Tbrake) > Tdead))
                %  --shift to PARK
                GEAR = 0;
            end
            
        elseif (gear_cmd == 1)
            %  --check to see if we can shift to DRIVE
            if ((abs(vc) <= Vdead) && (abs(Tbrake) > Tdead))
                %  --shift to DRIVE
                GEAR = 1;
            end
        end
        
    otherwise  %  --should never be here
        if (vc > Vdead)
            %  --moving forward, so must be in DRIVE
            GEAR = 1;
        elseif (vc < -Vdead)
            %  --moving backward, so must be in REVERSE
            GEAR = 2;
        else
            %  --vehicle stoppped, so must be in PARK
            GEAR = 0;
        end

end


%  --output the current actual gear setting

gear = GEAR;

return
